simulink model "nonUsedBlocks"  (R2023b)
settings: Solver=VariableStepAuto  StartTime=0.0  StopTime=10.0  RelTol=1e-3
undefined symbols (not defined in the file or in its folder): A_bar, AEFF, B_E, C_bar, C_T, Cd_neg, Cd_pos, DiscIntNeverNeededParam, Gamma, H, L_gain, L_STROKE, M, m3PsToLpm, P_return_Pa, P_supply_Pa, PA_Pa, PB_Pa, RHO, Ts, V01, V02, W
(part 2 of 2)

== matlab function nonUsedBlocks/old/Flow_Calc_WithLeak/MATLAB Function2 ==
  data: xv input; Q_A output; P_P input; P_T input; P_R input; P_A input; P_B input; w input; Q_B output; Q_Leak_Total_lpm output; c input; r input; rho input; mu input; Cd input; bias_P_dynamic input; bias_T_dynamic input; Q_return_model_lpm output; x_leak input
function [Q_A, Q_B, Q_Leak_Total_lpm, Q_return_model_lpm] = fcn_Valve_Tamburrano_Hybrid( ...
    xv, P_P, P_T, P_R, P_A, P_B, w, c, r, rho, mu, Cd, ...
    bias_P_dynamic, bias_T_dynamic, x_leak)

% SI units:
% xv [m], P_* [Pa], w,c,r [m], rho [kg/m^3], mu [Pa*s], Cd [-]
%
% Outputs:
%   Q_A, Q_B         : Port net flows [m^3/s]
%   Q_Leak_Total     : leakage indicator [m^3/s]
%   Q_return_lpm     : total return flow to return line [LPM]

%% 0) Checks
if c <= 0 || w <= 0 || rho <= 0 || mu <= 0 || Cd <= 0 || r < 0
    error('SI parametreler: w>0, c>0, r>=0, rho>0, mu>0, Cd>0 olmalı.');
end

%% 1) Tamburrano Eq.(19) -> l_eff (r,c'den)
if r == 0
    l_eff = c;
else
    y = (-(2*c + 4*r) + sqrt((2*c + 4*r)^2 + 16*r^2)) / 2; % y=l-c
    y = max(y, 0);
    l_eff = c + y;
end

%% 2) Tamburrano Eq.(18): laminer leakage conductance
K_lam_base = (pi * w * (l_eff^2)) / (32 * mu);  % [m^3/(s*Pa)]

%% 3) Static/Dynamic bias (pressure-holding + dynamic offset reduction)
transition_width = 20.5e-5;           % [m] (tune)
move_factor = tanh(abs(xv)/transition_width);

% --- Static
bias_P_static = 0.460;
bias_T_static = 0.9050;

% --- Interpolate to dynamic values ---
leak_bias_P = bias_P_static*(1-move_factor) + bias_P_dynamic*move_factor;
leak_bias_T = bias_T_static*(1-move_factor) + bias_T_dynamic*move_factor;


leak_bias_P = max(leak_bias_P, 0);
leak_bias_T = max(leak_bias_T, 0);



%% 4) Null-weighting for laminar leakage (keeps M-profile in motion)
% x_leak = 2.0e-4;                      % [m] (tune)
g = exp(-(abs(xv)/x_leak)^2);

%% 5) Metering areas
A_open = w * abs(xv);

if xv >= 0
    Area_PA = A_open;  Area_AT = 0;
    Area_PB = 0;       Area_BT = A_open;
else
    Area_PA = 0;       Area_AT = A_open;
    Area_PB = A_open;  Area_BT = 0;
end

%% 6) ΔP
dP_PA = (P_P - P_A);
dP_AT = (P_A - P_T);
dP_PB = (P_P - P_B);
dP_BT = (P_B - P_T);

%% 7) Orifice flows (Eq.7–10)
Q_PA_or = Cd * Area_PA * sign(dP_PA) * sqrt(2/rho * abs(dP_PA));
Q_AT_or = Cd * Area_AT * sign(dP_AT) * sqrt(2/rho * abs(dP_AT));
Q_PB_or = Cd * Area_PB * sign(dP_PB) * sqrt(2/rho * abs(dP_PB));
Q_BT_or = Cd * Area_BT * sign(dP_BT) * sqrt(2/rho * abs(dP_BT));

%% 8) Laminar leakage flows (Eq.18) with bias + null-weighting g
Q_PA_lam = (K_lam_base * leak_bias_P) * dP_PA;
Q_PB_lam = (K_lam_base * leak_bias_P) * dP_PB;
Q_AT_lam = (K_lam_base * leak_bias_T) * dP_AT;
Q_BT_lam = (K_lam_base * leak_bias_T) * dP_BT;

Q_PA = Q_PA_or + g * Q_PA_lam;
Q_PB = Q_PB_or + g * Q_PB_lam;
Q_AT = Q_AT_or + g * Q_AT_lam;
Q_BT = Q_BT_or + g * Q_BT_lam;

%% 9) Port net flows
Q_A = Q_PA - Q_AT;
Q_B = Q_PB - Q_BT;

%% 10) Return-line measured flow (valve-to-tank + extra bypass)
% Valve return to tank/return line:
Q_return_valve = max(Q_AT,0) + max(Q_BT,0);  % [m^3/s]

% C_bypass ≈ 6.43e-13 m^3/(s*Pa)
C_bypass = 6.43e-13; %1.628161 * 0.6*1.1;
Q_bypass = C_bypass * max(P_P - P_R, 0);     % [m^3/s]

Q_return_total = Q_return_valve + Q_bypass;
Q_return_model_lpm   = 60000 * Q_return_total;

%% 11) Leakage indicator (trend)
Q_Leak_Total = 0.5*(abs(Q_PA) + abs(Q_PB) + abs(Q_AT) + abs(Q_BT)) ...
              - 0.5*abs(Q_A + Q_B);
Q_Leak_Total_lpm = Q_Leak_Total * 60e3;
end

== matlab function nonUsedBlocks/Nguyen Observer/Nguyen_Observer/phi_calc/MATLAB Function ==
  data: Q1 output; Q2 output; u input; Ps input; Pr input; P1 input; P2 input; QR output
function [Q1, Q2, QR] = fcn(u, Ps, Pr, P1, P2)
    % x0 parametresini girişten kaldırdık, içeride asimetrik tanımlayacağız.
    % Valve params 
    K           = 0.00000334; 
    k           = 1.82709080; 

    % --- ASİMETRİK SIZINTI AYARLARI ---
    % Hedef: P_null = 70 bar (Ps=210 bar iken)
    % Bu dengeyi sağlamak için Return tarafı açıklığı daha büyük olmalı.

    % --- GÜNCELLENMİŞ ASİMETRİK SIZINTI AYARLARI ---
    % Hedef: Ps=200 bar, Pr=4.5 bar iken yaklaşık 70-75 bar denge basıncı
    % $$x_{0S} \cdot \sqrt{130} = x_{0R} \cdot \sqrt{70}$$ --> Ortalamaları
    % da bulunan x0 olacak.

    % Ortalama x0 = 0.53e-3 idi. Bunu asimetrik dağıtıyoruz:
    % x0_S = 0.47e-3;  % Supply tarafı (0.47 mA)
    % x0_R = 0.64e-3;  % Return tarafı (0.64 mA)
    
    x0_S = 0.46e-3 ;  % Supply tarafı (0.46 mA) --> bunu editledim
    x0_R = 0.64e-3 ;  % Return tarafı (0.64 mA)

    % x0_S = 0.53e-3;  % Supply tarafı (0.47 mA)
    % x0_R = 0.53e-3;  % Return tarafı (0.64 mA)

    K_tare = 2.345e-9; 
    
    % Güvenlik (Basınçlar)
    dPs1 = max(0, Ps - P1); dP1r = max(0, P1 - Pr);
    dPs2 = max(0, Ps - P2); dP2r = max(0, P2 - Pr);
    dPsr = max(0, Ps - Pr);

    if u >= 0
        % P_S -> P_1 (Supply Side - Ana Akış) -> x0_S kullan
        Q1_S = K * sqrt(dPs1) * (x0_S + u); 
        
        % P_1 -> P_R (Return Side - Sızıntı) -> x0_R kullan
        Q1_R = K * sqrt(dP1r) * (x0_R^2 / (x0_R + k*u)); 

        % P_S -> P_2 (Supply Side - Sızıntı) -> x0_S kullan
        Q2_S = K * sqrt(dPs2) * (x0_S^2 / (x0_S + k*u)); 
        
        % P_2 -> P_R (Return Side - Ana Akış) -> x0_R kullan
        Q2_R = K * sqrt(dP2r) * (x0_R + u);
    else
        % x < 0 durumu
        % Simetriyi korumak için x negatifken de Supply/Return rollerine göre
        % doğru x0'ı seçmeliyiz.
        
        % P_S -> P_1 (Supply Side - Sızıntı)
        Q1_S = K * sqrt(dPs1) * (x0_S^2 / (x0_S - k*u)); 
        
        % P_1 -> P_R (Return Side - Ana Akış)
        Q1_R = K * sqrt(dP1r) * (x0_R - u); 

        % P_S -> P_2 (Supply Side - Ana Akış)
        Q2_S = K * sqrt(dPs2) * (x0_S - u); 
        
        % P_2 -> P_R (Return Side - Sızıntı)
        Q2_R = K * sqrt(dP2r) * (x0_R^2 / (x0_R - k*u)); 
    end

    Q1 = Q1_S - Q1_R;
    Q2 = Q2_S - Q2_R;
    QR = Q1_R + (Q2_R) + K_tare * sqrt(dPsr); 
end

== matlab function nonUsedBlocks/Nguyen Observer/Nguyen_Observer/phi_calc/MATLAB Function4 ==
  data: v input; F_stribeck output
function F_stribeck = fcn(v)


% close all 

% --- Geçiş Yumuşaklığı Parametresi ---
% Bu değer büyüdükçe 0'daki eğim azalır (daha eğimli geçer)
eps_smooth = 0.0223;
% eps_smooth = 0.015;

%%%
kv_p = 12; Fc_p = 25; Fs_p  = 383; tau_p = 0.016;
kv_n = 35; Fc_n = 7.5; Fs_n = 183; tau_n = 0.02016;
%%%


% Yumuşatılmış yön fonksiyonu (sign yerine tanh)
% Bu fonksiyon -1 ile 1 arasında yumuşak bir geçiş sağlar
smooth_sign = tanh(v ./ eps_smooth);

% Asimetrik katsayı vektörleri oluşturma
% Hızın yönüne göre katsayıları seçiyoruz
kv = (v >= 0)*kv_p + (v < 0)*kv_n;
Fc = (v >= 0)*Fc_p + (v < 0)*Fc_n;
Fs = (v >= 0)*Fs_p + (v < 0)*Fs_n;
tau = (v >= 0)*tau_p + (v < 0)*tau_n;
F_stribeck = (Fc .* smooth_sign) + (Fs .* smooth_sign .* exp(-abs(v./tau)));

== matlab function nonUsedBlocks/LinModel ==
  data: u input; f input; x input; xdot output
function xdot = hydraulic_plant_3states(u, f, x)
    % Makaledeki Denklem (9)'a göre 3 Durumlu Hidrolik Sistem Modeli
    % GİRİŞLER:
    % x(1) : Piston konumu (x_p) [m]
    % x(2) : Piston hızı (\dot{x}_p) [m/s]
    % x(3) : Yük basıncı (P_L) [Pa]
    % u    : Kontrol sinyali (Valf giriş gerilimi) [V]
    % f    : Modellenmemiş sürtünme ve dış bozucular [N]

    % PARAMETRELER 
    d_p     = 34e-3;
    d_r     = 30e-3;
    A_c     = pi/4*(d_p^2 - d_r^2);
    V_dead  = 1.5315e-5;
    V_0     = A_c*(190.16e-3/2) + V_dead;
    
    m      = 3.4;                   % Piston rotu eşdeğer kütlesi [kg]
    Ae     = A_c;                   % Efektif alan [m^2] (Çift kollu silindirde doğrudan A'ya eşittir)
    Bp     = 38;                    % Viskoz sönümleme katsayısı [N/(m/s)]
    beta_e = 1.6e9;                 % Hidrolik yağın efektif elastikiyet (bulk) modülü [Pa]
    Ve     = 2*V_0;                 % Efektif hacim [m^3]
    Kq     = 1.1003e-2;              % Akış kazancı [(m^3/s)/m]
    Kv     = 1;                     % Servo valf spool kazancı [m/V]
    Kc     = 3.9633e-13; %3.9633e-13;            % Basınç-akış katsayısı [(m^3/s)/Pa]
    Cip    = 3.9933e-13;            % Silindir içi kaçak katsayısı [(m^3/s)/Pa]

    % Durum değişkenlerini okuma
    x1 = x(1); % x_p
    x2 = x(2); % \dot{x}_p
    x3 = x(3); % P_L

    % Denklem 9: Durum uzayı türevlerinin (State derivatives) hesaplanması
    x1_dot = x2;
    x2_dot = (-Ae * x3 - Bp * x2 - f) / m;
    x3_dot = (4 * beta_e / Ve) * (-Kq * Kv *u - (Kc + Cip) * x3 + Ae * x2); % u teriminin önüne eksi (-) geldi

    % Çıkış vektörünü oluşturma (Sütun vektörü olmalıdır)
    xdot = [x1_dot; x2_dot; x3_dot];
end
